simulink model "nid_cvst_skeleton"  (Simulink 7.6)
settings: Solver=FixedStepDiscrete  StartTime=0.0  StopTime=inf  RelTol=1e-3
undefined symbols (not defined in the file): jet
libraries: vipsnks x2, nid_lib x2
settings Model: Creator=tchikama  LastModifiedBy=tchikama
settings DataIOCC: SaveOutput=off
settings OptimizationCC: SimCompilerOptimization=On
settings HardwareCC: ProdIntDivRoundTo=Zero  ProdEndianess=LittleEndian  ProdHWDeviceType=Generic->32-bit x86 compatible
settings RTWCC: ProcessScript=grt_make_rtw_hook  RTWCompilerOptimization=On
settings CodeAppCC: MaxIdLength=95

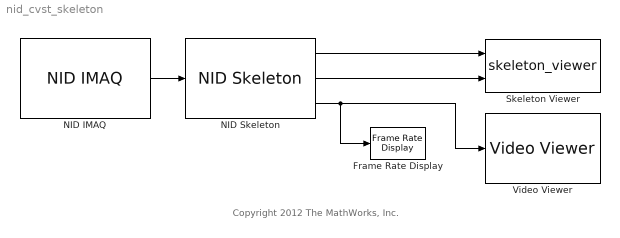
== system nid_cvst_skeleton ==
  note: Copyright 2012 The MathWorks, Inc.
  Frame Rate Display : vipsnks/Frame Rate Display  DialogController=vipDDGCreate  DialogControllerArgs=DataTag0  UpdateRate=10
  NID IMAQ : nid_lib/NID IMAQ  imaq_depth=off  imaq_motion=off  imaq_image=off  view_point=off  imaq_skeleton=on  imaq_ir=off  mirror_image=off  imaq_sample_time=1/30  res_fps=VGA (640x480): 30 FPS  needPsiPose=off  angle=0  angle_read=off  near_mode=off  seated_mode=off
  NID Skeleton : nid_lib/NID Skeleton  num_of_skeleton_tracking=1  conv_XYZ_RW=on  viewer=on
  Skeleton Viewer : M-S-Function  FunctionName=skeleton_viewer
      mask Display:
      | disp('Skeleton\nViewer')
      | 
      | port_label('input', 1, 'Tracking')
      | port_label('input', 2, 'Skeleton')
  Video Viewer : vipsnks/Video Viewer  DialogControllerArgs=DataTag2  inputType=Obsolete7b  imagePorts=One multidimensional signal  useColorMap=off  colormapValue=jet(256)  specRange=off  minInputVal=0  maxInputVal=255  FigPos=[755 749 410 300]  AxisZoom=on  trueSizedOnce=off  OpenAtMdlStart=on
  wires:
  NID IMAQ/1 -> NID Skeleton/1
  NID Skeleton/1 -> Skeleton Viewer/1
  NID Skeleton/2 -> Skeleton Viewer/2
  NID Skeleton/3 -> Frame Rate Display/1, Video Viewer/1
